simulink subsystem "SubSystemBefullung"  (R2020b)
settings: Solver=VariableStepAuto  StartTime=0.0  StopTime=10.0  RelTol=1e-3
libraries: simulink x2
settings Model: Creator=kaebi  LastModifiedBy=kaebi

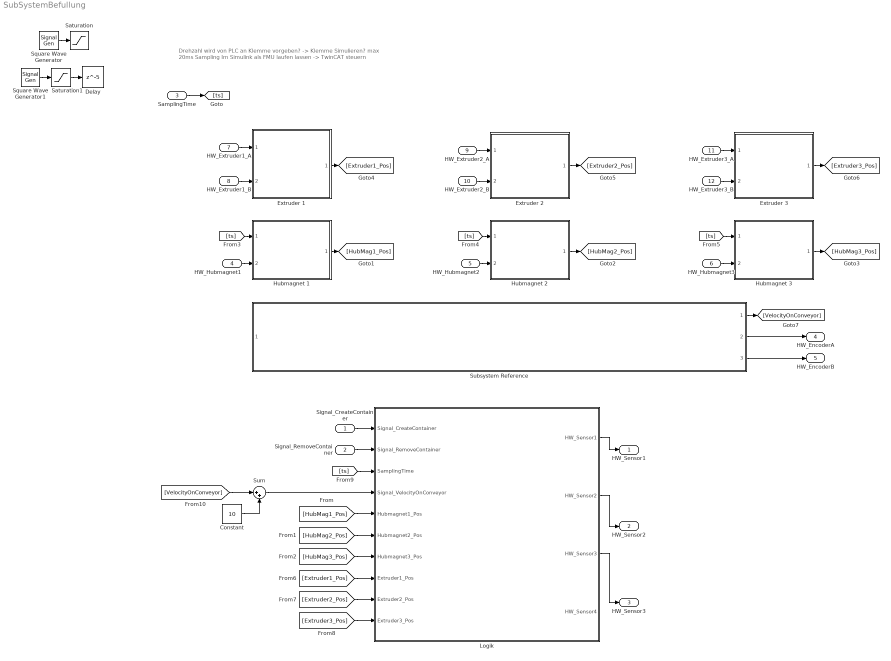
== system SubSystemBefullung ==
  note: Drehzahl wird von PLC an Klemme vorgeben? -> Klemme Simulieren?
      |
      | max 20ms Sampling
      | Im Simulink als FMU laufen lassen -> TwinCAT steuern
  Signal_CreateContainer : Inport
  Signal_RemoveContainer : Inport  Port=2
  SamplingTime : Inport  Port=3
  HW_Hubmagnet1 : Inport  Port=4
  HW_Hubmagnet2 : Inport  Port=5
  HW_Hubmagnet3 : Inport  Port=6
  HW_Extruder1_A : Inport  Port=7
  HW_Extruder1_B : Inport  Port=8
  HW_Extruder2_A : Inport  Port=9
  HW_Extruder2_B : Inport  Port=10
  HW_Extruder3_A : Inport  Port=11
  HW_Extruder3_B : Inport  Port=12
  Constant : Constant  Value=10
  Delay : Delay  DelayLength=5
  Extruder 1 : Subsystem  ReferencedSubsystem=SubSystemExtruder
  Extruder 2 : Subsystem  ReferencedSubsystem=SubSystemExtruder
  Extruder 3 : Subsystem  ReferencedSubsystem=SubSystemExtruder
  Hubmagnet 1 : Subsystem  ReferencedSubsystem=SubSystemHubmagnetConveyor
  Hubmagnet 2 : Subsystem  ReferencedSubsystem=SubSystemHubmagnetConveyor
  Hubmagnet 3 : Subsystem  ReferencedSubsystem=SubSystemHubmagnetConveyor
  Logik : Subsystem
  Saturation : Saturate  UpperLimit=1  LowerLimit=0
  Saturation1 : Saturate  UpperLimit=1  LowerLimit=0
  Square Wave Generator : SignalGenerator  WaveForm=square  Frequency=100
  Square Wave Generator1 : SignalGenerator  WaveForm=square  Frequency=100
  Subsystem Reference : Subsystem  ReferencedSubsystem=SubSystemMotorConveyor
  Sum : Sum  Inputs=|++
  HW_Sensor1 : Outport
  HW_Sensor2 : Outport  Port=2
  HW_Sensor3 : Outport  Port=3
  HW_EncoderA : Outport  Port=4
  HW_EncoderB : Outport  Port=5
  wires:
  SamplingTime/1 -> [ts]
  Subsystem Reference/3 -> HW_EncoderB/1
  Subsystem Reference/2 -> HW_EncoderA/1
  Logik/1(HW_Sensor1) -> HW_Sensor1/1
  Logik/2(HW_Sensor2) -> HW_Sensor2/1
  Logik/3(HW_Sensor3) -> HW_Sensor3/1
  Hubmagnet 1/1 -> [HubMag1_Pos]
  Hubmagnet 2/1 -> [HubMag2_Pos]
  Hubmagnet 3/1 -> [HubMag3_Pos]
  [HubMag1_Pos] -> Logik/5(Hubmagnet1_Pos)
  [HubMag2_Pos] -> Logik/6(Hubmagnet2_Pos)
  [HubMag3_Pos] -> Logik/7(Hubmagnet3_Pos)
  HW_Hubmagnet1/1 -> Hubmagnet 1/2
  HW_Hubmagnet2/1 -> Hubmagnet 2/2
  HW_Hubmagnet3/1 -> Hubmagnet 3/2
  [ts] -> Hubmagnet 1/1
  [ts] -> Hubmagnet 2/1
  [ts] -> Hubmagnet 3/1
  Signal_RemoveContainer/1 -> Logik/2(Signal_RemoveContainer)
  Signal_CreateContainer/1 -> Logik/1(Signal_CreateContainer)
  Square Wave Generator/1 -> Saturation/1
  Square Wave Generator1/1 -> Saturation1/1
  Saturation1/1 -> Delay/1
  HW_Extruder1_A/1 -> Extruder 1/1
  HW_Extruder1_B/1 -> Extruder 1/2
  HW_Extruder2_B/1 -> Extruder 2/2
  HW_Extruder2_A/1 -> Extruder 2/1
  HW_Extruder3_A/1 -> Extruder 3/1
  HW_Extruder3_B/1 -> Extruder 3/2
  Extruder 2/1 -> [Extruder2_Pos]
  Extruder 1/1 -> [Extruder1_Pos]
  Extruder 3/1 -> [Extruder3_Pos]
  [Extruder1_Pos] -> Logik/8(Extruder1_Pos)
  [Extruder2_Pos] -> Logik/9(Extruder2_Pos)
  [Extruder3_Pos] -> Logik/10(Extruder3_Pos)
  [ts] -> Logik/3(SamplingTime)
  Subsystem Reference/1 -> [VelocityOnConveyor]
  [VelocityOnConveyor] -> Sum/1
  Sum/1 -> Logik/4(Signal_VelocityOnConveyor)
  Constant/1 -> Sum/2

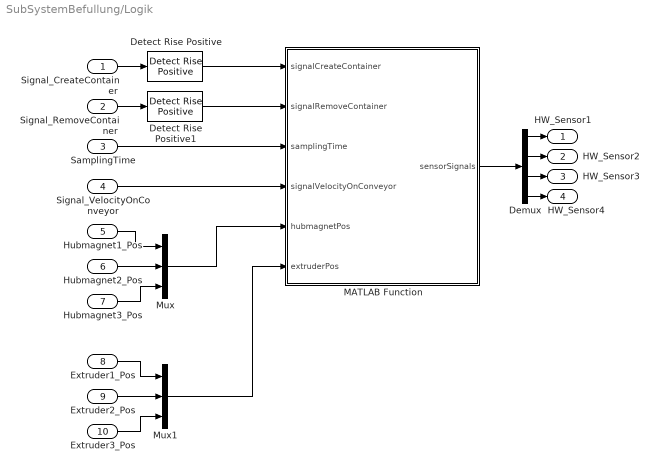
== system SubSystemBefullung/Logik ==
  Signal_CreateContainer : Inport
  Signal_RemoveContainer : Inport  Port=2
  SamplingTime : Inport  Port=3
  Signal_VelocityOnConveyor : Inport  Port=4
  Hubmagnet1_Pos : Inport  Port=5
  Hubmagnet2_Pos : Inport  Port=6
  Hubmagnet3_Pos : Inport  Port=7
  Extruder1_Pos : Inport  Port=8
  Extruder2_Pos : Inport  Port=9
  Extruder3_Pos : Inport  Port=10
  Demux : Demux
  Detect Rise Positive : simulink/Logic and Bit Operations/Detect Rise Positive  vinit=0  OutDataTypeStr=boolean
  Detect Rise Positive1 : simulink/Logic and Bit Operations/Detect Rise Positive  vinit=0  OutDataTypeStr=boolean
  MATLAB Function : MATLAB Function  TreatAsAtomicUnit=on
  Mux : Mux  Inputs=3
  Mux1 : Mux  Inputs=3
  HW_Sensor1 : Outport
  HW_Sensor2 : Outport  Port=2
  HW_Sensor3 : Outport  Port=3
  HW_Sensor4 : Outport  Port=4
  wires:
  Demux/4 -> HW_Sensor4/1
  Detect Rise Positive1/1 -> MATLAB Function/2(signalRemoveContainer)
  Detect Rise Positive/1 -> MATLAB Function/1(signalCreateContainer)
  Demux/3 -> HW_Sensor3/1
  Demux/2 -> HW_Sensor2/1
  Demux/1 -> HW_Sensor1/1
  MATLAB Function/1(sensorSignals) -> Demux/1
  Mux1/1 -> MATLAB Function/6(extruderPos)
  Mux/1 -> MATLAB Function/5(hubmagnetPos)
  Signal_VelocityOnConveyor/1 -> MATLAB Function/4(signalVelocityOnConveyor)
  SamplingTime/1 -> MATLAB Function/3(samplingTime)
  Signal_RemoveContainer/1 -> Detect Rise Positive1/1
  Signal_CreateContainer/1 -> Detect Rise Positive/1
  Extruder3_Pos/1 -> Mux1/3
  Extruder1_Pos/1 -> Mux1/1
  Extruder2_Pos/1 -> Mux1/2
  Hubmagnet3_Pos/1 -> Mux/3
  Hubmagnet2_Pos/1 -> Mux/2
  Hubmagnet1_Pos/1 -> Mux/1

== matlab function SubSystemBefullung/Logik/MATLAB Function ==
  settings: updateMethod=DISCRETE
  data: signalCreateContainer input; sensorSignals output; signalRemoveContainer input; samplingTime input; signalVelocityOnConveyor input; hubmagnetPos input; extruderPos input
function sensorSignals = fcn(signalCreateContainer, signalRemoveContainer, samplingTime, signalVelocityOnConveyor, hubmagnetPos, extruderPos)
    % samplingTime in s
    % signalVelocityOnConveyor in mm/s
    % hubmagnetPos between 1 () and 0 ()
    
    %% Mechanical Properties
    posStopperOnConveyor = [100 200 300 400]';
    posEndOfConveyor = 400;
    
    %%  Variables
    persistent containers                   % Store Position in mm
    persistent containersValid
    sensorSignals = [false, false, false, false]';
    stopperStatePassable = [hubmagnetPos; 0];       % 0=Stopping
    
    if (isempty(containersValid))
        containersValid = false;
    end
    
    if (isempty(containers))
        containers = [0];
    end
    
    %% Create Container on Signal
    if (signalCreateContainer == true)
        if (containersValid == false)
            containersValid = true;
        else
            containers = [containers 0];
        end
    end
    
    %% Remove Container On Signal
    if (signalRemoveContainer==true)
        if (max(size(containers)) > 1)
            containers(1) = [];
        else
            containersValid = false;
        end
    end
    
    %% Logic
    travelDistance = signalVelocityOnConveyor*samplingTime;
    if (containersValid == true)
        for idxContainer = 1:max(size(containers))
            containerPos = containers(idxContainer);
            
            for idxStopper = 1:max(size(posStopperOnConveyor))
                if (containerPos < posStopperOnConveyor(idxStopper))
                    distanceToStopper = posStopperOnConveyor(idxStopper)-containerPos;
                    
                    % Stop before stopper
                    if (stopperStatePassable(idxStopper) == false && containerPos+travelDistance >= distanceToStopper)
                        travelDistance = distanceToStopper-1;
                    end                    
                    
                    % Set Sensor if needed
                    if (distanceToStopper < 3)                    
                        sensorSignals(idxStopper) = true;
                    end
                    
                    break;
                end                    
            end    
            
            % Change position of container if possible
            containers(idxContainer) = containers(idxContainer) + travelDistance;
        end        
    end
end
